simulink model "RC_buttom_Evaporator_1"  (R2018b)
settings: Solver=VariableStepAuto  StartTime=0.0  StopTime=500000.0  RelTol=1e-3
settings Model: Creator=user  LastModifiedBy=user

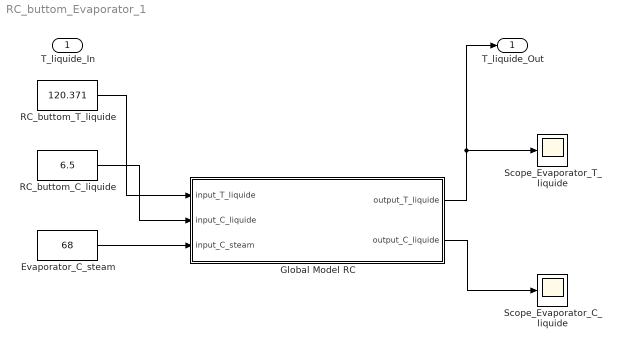
== system RC_buttom_Evaporator_1 ==
  T_liquide_In : Inport
  Evaporator_C_steam : Constant  Value=68
  Global Model RC : Subsystem
  RC_buttom_C_liquide : Constant  Value=6.5
  RC_buttom_T_liquide : Constant  Value=120.371
  Scope_Evaporator_C_liquide : Scope
  Scope_Evaporator_T_liquide : Scope
  T_liquide_Out : Outport
  wires:
  Global Model RC/1(output_T_liquide) -> T_liquide_Out/1, Scope_Evaporator_T_liquide/1
  Global Model RC/2(output_C_liquide) -> Scope_Evaporator_C_liquide/1
  Evaporator_C_steam/1 -> Global Model RC/3(input_C_steam)
  RC_buttom_C_liquide/1 -> Global Model RC/2(input_C_liquide)
  RC_buttom_T_liquide/1 -> Global Model RC/1(input_T_liquide)

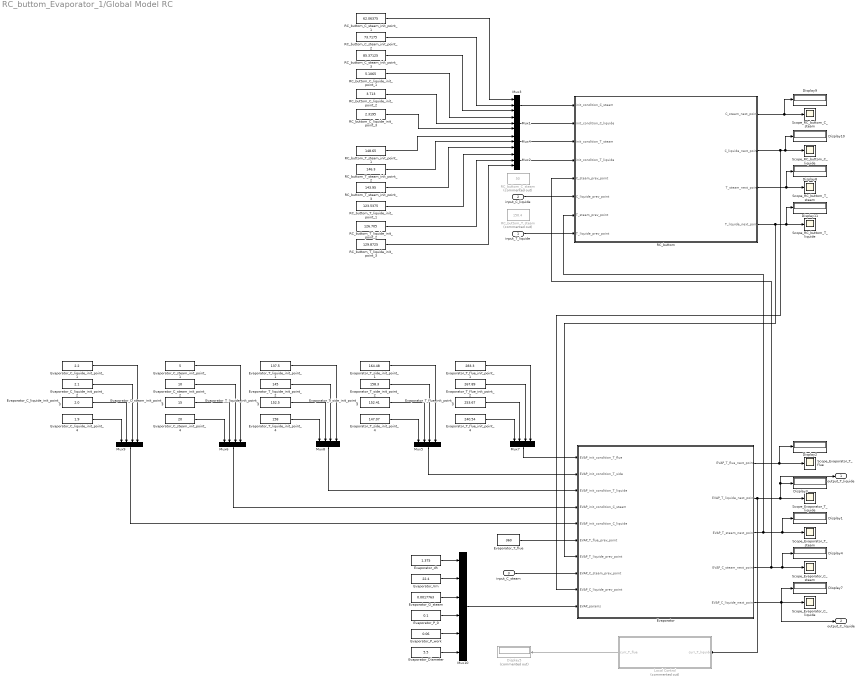
== system RC_buttom_Evaporator_1/Global Model RC ==
  input_T_liquide : Inport
  input_C_liquide : Inport  Port=2
  input_C_steam : Inport  Port=3
  Display{1..4,7..11} (9 alike) : Display
  Display5 : Display  Commented=on
  Evaporator : Subsystem
  Evaporator_C_liquide_init_point_1 : Constant  Value=2.2
  Evaporator_C_liquide_init_point_2 : Constant  Value=2.1
  Evaporator_C_liquide_init_point_3 : Constant  Value=2.0
  Evaporator_C_liquide_init_point_4 : Constant  Value=1.9
  Evaporator_C_steam_init_point_1 : Constant  Value=5
  Evaporator_C_steam_init_point_2 : Constant  Value=10
  Evaporator_C_steam_init_point_3 : Constant  Value=15
  Evaporator_C_steam_init_point_4 : Constant  Value=20
  Evaporator_Diameter : Constant  Value=5.5
  Evaporator_G_steam : Constant  Value=0.0017763
  Evaporator_P_0 : Constant  Value=0.1
  Evaporator_P_work : Constant  Value=0.06
  Evaporator_T_flue : Constant  Value=360
  Evaporator_T_flue_init_point_1 : Constant  Value=283.3
  Evaporator_T_flue_init_point_2 : Constant  Value=267.89
  Evaporator_T_flue_init_point_3 : Constant  Value=253.67
  Evaporator_T_flue_init_point_4 : Constant  Value=240.54
  Evaporator_T_liquide_init_point_1 : Constant  Value=137.5
  Evaporator_T_liquide_init_point_2 : Constant  Value=145
  Evaporator_T_liquide_init_point_3 : Constant  Value=152.5
  Evaporator_T_liquide_init_point_4 : Constant  Value=158
  Evaporator_T_side_init_point_1 : Constant  Value=164.48
  Evaporator_T_side_init_point_2 : Constant  Value=158.3
  Evaporator_T_side_init_point_3 : Constant  Value=152.41
  Evaporator_T_side_init_point_4 : Constant  Value=147.07
  Evaporator_Vm : Constant  Value=22.4
  Evaporator_dh : Constant  Value=1.375
  Local Control : Subsystem  Commented=on
  Mux{1..4} (4 alike) : Mux  Inputs=3
  Mux10 : Mux  Inputs=6
  Mux{5..9} (5 alike) : Mux
  RC_buttom : Subsystem
  RC_buttom_C_liquide_init_point_1 : Constant  Value=5.1065
  RC_buttom_C_liquide_init_point_2 : Constant  Value=3.713
  RC_buttom_C_liquide_init_point_3 : Constant  Value=2.3195
  RC_buttom_C_steam : Constant  Commented=on  Value=50
  RC_buttom_C_steam_init_point_1 : Constant  Value=62.06375
  RC_buttom_C_steam_init_point_2 : Constant  Value=73.7175
  RC_buttom_C_steam_init_point_3 : Constant  Value=85.37125
  RC_buttom_T_liquide_init_point_1 : Constant  Value=123.5375
  RC_buttom_T_liquide_init_point_2 : Constant  Value=126.705
  RC_buttom_T_liquide_init_point_3 : Constant  Value=129.8725
  RC_buttom_T_steam : Constant  Commented=on  Value=150.4
  RC_buttom_T_steam_init_point_1 : Constant  Value=148.65
  RC_buttom_T_steam_init_point_2 : Constant  Value=146.3
  RC_buttom_T_steam_init_point_3 : Constant  Value=143.95
  Scope_Evaporator_C_liquide : Scope
  Scope_Evaporator_C_steam : Scope
  Scope_Evaporator_T_flue : Scope
  Scope_Evaporator_T_liquide : Scope
  Scope_Evaporator_T_steam : Scope
  Scope_RC_buttom_C_liquide : Scope
  Scope_RC_buttom_C_steam : Scope
  Scope_RC_buttom_T_liquide : Scope
  Scope_RC_buttom_T_steam : Scope
  output_T_liquide : Outport
  output_C_liquide : Outport  Port=2
  wires:
  Evaporator_T_side_init_point_3/1 -> Mux5/2
  Evaporator_C_steam_init_point_2/1 -> Mux6/3
  Evaporator_C_liquide_init_point_1/1 -> Mux9/4
  RC_buttom_T_steam_init_point_1/1 -> Mux4/1
  Evaporator_C_steam_init_point_4/1 -> Mux6/1
  RC_buttom_C_steam_init_point_1/1 -> Mux3/1
  Mux1/1 -> RC_buttom/2(init_condition_C_liquide)
  Evaporator_T_liquide_init_point_4/1 -> Mux8/1
  Evaporator_C_steam_init_point_3/1 -> Mux6/2
  Evaporator/2(EVAP_T_liquide_next_point) -> Local Control/1(curr_T_liquide), output_T_liquide/1, Display3/1, Scope_Evaporator_T_liquide/1
  RC_buttom/4(T_liquide_next_point) -> Evaporator/7(EVAP_T_liquide_prev_point), Display11/1, Scope_RC_buttom_T_liquide/1
  Evaporator_C_liquide_init_point_2/1 -> Mux9/3
  Evaporator_G_steam/1 -> Mux10/3
  Local Control/1(curr_T_flue) -> Display5/1
  Mux8/1 -> Evaporator/3(EVAP_init_condition_T_liquide)
  Evaporator_P_0/1 -> Mux10/4
  Mux6/1 -> Evaporator/4(EVAP_init_condition_C_steam)
  Evaporator_T_flue_init_point_2/1 -> Mux7/3
  RC_buttom_C_liquide_init_point_2/1 -> Mux1/2
  Evaporator_P_work/1 -> Mux10/5
  RC_buttom_T_steam_init_point_3/1 -> Mux4/3
  Evaporator_C_liquide_init_point_3/1 -> Mux9/2
  Evaporator_C_liquide_init_point_4/1 -> Mux9/1
  input_T_liquide/1 -> RC_buttom/8(T_liquide_prev_point)
  Mux4/1 -> RC_buttom/3(init_condition_T_steam)
  Evaporator/1(EVAP_T_flue_next_point) -> Display2/1, Scope_Evaporator_T_flue/1
  Evaporator_T_flue_init_point_4/1 -> Mux7/1
  RC_buttom/3(T_steam_next_point) -> Display8/1, Scope_RC_buttom_T_steam/1
  Evaporator/3(EVAP_T_steam_next_point) -> Display1/1, Scope_Evaporator_T_steam/1, RC_buttom/7(T_steam_prev_point)
  RC_buttom_C_liquide_init_point_1/1 -> Mux1/1
  Evaporator_T_flue_init_point_1/1 -> Mux7/4
  RC_buttom/2(C_liquide_next_point) -> Display10/1, Scope_RC_buttom_C_liquide/1, Evaporator/9(EVAP_C_liquide_prev_point)
  Evaporator/5(EVAP_C_liquide_next_point) -> output_C_liquide/1, Display7/1, Scope_Evaporator_C_liquide/1
  Mux3/1 -> RC_buttom/1(init_condition_C_steam)
  Evaporator_T_side_init_point_1/1 -> Mux5/4
  RC_buttom_T_steam_init_point_2/1 -> Mux4/2
  RC_buttom_C_steam_init_point_2/1 -> Mux3/2
  Evaporator_T_side_init_point_2/1 -> Mux5/3
  RC_buttom_T_liquide_init_point_1/1 -> Mux2/1
  Evaporator_T_side_init_point_4/1 -> Mux5/1
  Evaporator_T_flue_init_point_3/1 -> Mux7/2
  RC_buttom_C_liquide_init_point_3/1 -> Mux1/3
  Evaporator_T_liquide_init_point_1/1 -> Mux8/4
  RC_buttom_T_liquide_init_point_3/1 -> Mux2/3
  RC_buttom/1(C_steam_next_point) -> Display9/1, Scope_RC_buttom_C_steam/1
  Evaporator_T_liquide_init_point_2/1 -> Mux8/3
  Evaporator_Vm/1 -> Mux10/2
  Mux7/1 -> Evaporator/1(EVAP_init_condition_T_flue)
  RC_buttom_T_liquide_init_point_2/1 -> Mux2/2
  Mux5/1 -> Evaporator/2(EVAP_init_condition_T_side)
  input_C_steam/1 -> Evaporator/8(EVAP_C_steam_prev_point)
  Mux2/1 -> RC_buttom/4(init_condition_T_liquide)
  Evaporator/4(EVAP_C_steam_next_point) -> RC_buttom/5(C_steam_prev_point), Display4/1, Scope_Evaporator_C_steam/1
  Mux10/1 -> Evaporator/10(EVAP_params)
  Evaporator_C_steam_init_point_1/1 -> Mux6/4
  Evaporator_T_liquide_init_point_3/1 -> Mux8/2
  Mux9/1 -> Evaporator/5(EVAP_init_condition_C_liquide)
  RC_buttom_C_steam_init_point_3/1 -> Mux3/3
  Evaporator_dh/1 -> Mux10/1
  Evaporator_Diameter/1 -> Mux10/6
  input_C_liquide/1 -> RC_buttom/6(C_liquide_prev_point)
  Evaporator_T_flue/1 -> Evaporator/6(EVAP_T_flue_prev_point)

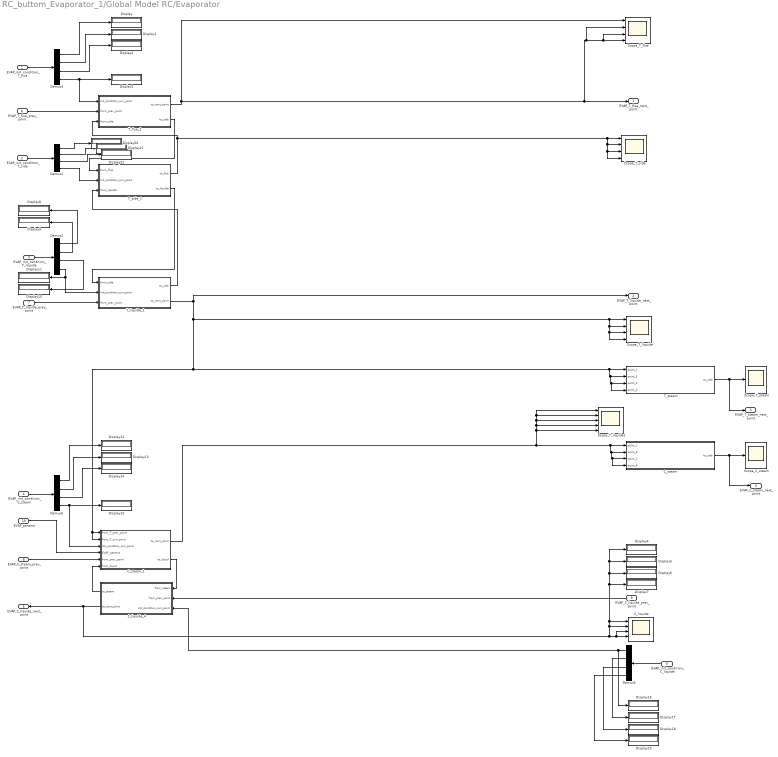
== system RC_buttom_Evaporator_1/Global Model RC/Evaporator ==
  EVAP_init_condition_T_flue : Inport
  EVAP_init_condition_T_side : Inport  Port=2
  EVAP_init_condition_T_liquide : Inport  Port=3
  EVAP_init_condition_C_steam : Inport  Port=4
  EVAP_init_condition_C_liquide : Inport  Port=5
  EVAP_T_flue_prev_point : Inport  Port=6
  EVAP_T_liquide_prev_point : Inport  Port=7
  EVAP_C_steam_prev_point : Inport  Port=8
  EVAP_C_liquide_prev_point : Inport  Port=9
  EVAP_params : Inport  Port=10
  C_liquide : Scope  NumInputPorts=4
  C_liquide_4 : Subsystem
  C_steam : Subsystem
  C_steam_1 : Subsystem
  Demux{1..5} (5 alike) : Demux
  Display{,1..22} (23 alike) : Display
  Scope_C_steam : Scope
  Scope_T_flue : Scope  NumInputPorts=4
  Scope_T_liquide : Scope  NumInputPorts=4
  Scope_T_liquide1 : Scope  NumInputPorts=5
  Scope_T_side : Scope  NumInputPorts=4
  Scope_T_steam : Scope
  T_flue_1 : Subsystem
  T_liquide_1 : Subsystem
  T_side_1 : Subsystem
  T_steam : Subsystem
  EVAP_T_flue_next_point : Outport
  EVAP_T_liquide_next_point : Outport  Port=2
  EVAP_T_steam_next_point : Outport  Port=3
  EVAP_C_steam_next_point : Outport  Port=4
  EVAP_C_liquide_next_point : Outport  Port=5
  wires:
  EVAP_init_condition_T_liquide/1 -> Demux2/1
  Demux2/1 -> Display8/1
  EVAP_init_condition_T_side/1 -> Demux1/1
  Demux2/2 -> Display9/1
  Demux2/4 -> T_liquide_1/2(init_condition_curr_point), Display11/1
  EVAP_init_condition_T_flue/1 -> Demux3/1
  Demux3/1 -> Display/1
  Demux3/2 -> Display1/1
  Demux3/3 -> Display2/1
  Demux3/4 -> T_flue_1/1(init_condition_curr_point), Display3/1
  T_flue_1/1(to_next_point) -> EVAP_T_flue_next_point/1, Scope_T_flue/2, Scope_T_flue/3, Scope_T_flue/4, Scope_T_flue/1
  EVAP_T_flue_prev_point/1 -> T_flue_1/2(from_prev_point)
  T_steam/1(to_side) -> EVAP_T_steam_next_point/1, Scope_T_steam/1
  Demux5/2 -> Display13/1
  EVAP_init_condition_C_liquide/1 -> Demux4/1
  Demux5/3 -> Display14/1
  C_steam_1/2(to_liquid) -> C_liquide_4/1(from_steam)
  Demux5/1 -> Display12/1
  EVAP_init_condition_C_steam/1 -> Demux5/1
  EVAP_C_steam_prev_point/1 -> C_steam_1/5(from_prev_point)
  C_liquide_4/2(to_next_point) -> EVAP_C_liquide_next_point/1, C_liquide/2, C_liquide/1, Display6/1, Display5/1, Display4/1, Display7/1, C_liquide/3, C_liquide/4
  EVAP_C_liquide_prev_point/1 -> C_liquide_4/2(from_prev_point)
  C_liquide_4/1(to_steam) -> C_steam_1/6(from_liquid)
  Demux5/4 -> C_steam_1/3(init_condition_curr_point), Display15/1
  Demux4/1 -> C_liquide_4/3(init_condition_curr_point), Display16/1
  Demux4/2 -> Display17/1
  Demux4/3 -> Display18/1
  Demux4/4 -> Display19/1
  C_steam/1(to_side) -> EVAP_C_steam_next_point/1, Scope_C_steam/1
  EVAP_params/1 -> C_steam_1/4(EVAP_params)
  EVAP_T_liquide_prev_point/1 -> T_liquide_1/3(from_prev_point)
  Demux2/3 -> Display10/1
  T_flue_1/2(to_side) -> T_side_1/1(from_flue)
  T_side_1/2(to_liquide) -> T_liquide_1/1(from_side)
  T_liquide_1/1(to_side) -> T_side_1/3(from_liquide)
  Demux1/4 -> T_side_1/2(init_condition_curr_point)
  T_side_1/1(to_flue) -> Scope_T_side/4, Scope_T_side/3, Scope_T_side/2, Scope_T_side/1, T_flue_1/3(from_side)
  Demux1/1 -> Display20/1
  Demux1/2 -> Display21/1
  Demux1/3 -> Display22/1
  T_liquide_1/2(to_next_point) -> EVAP_T_liquide_next_point/1, Scope_T_liquide/4, Scope_T_liquide/3, Scope_T_liquide/2, Scope_T_liquide/1, T_steam/4(point_4), T_steam/3(point_2), T_steam/2(point_3), T_steam/1(point_1), C_steam_1/1(from_T_prev_point), C_steam_1/2(from_T_curr_point)
  C_steam_1/1(to_next_point) -> Scope_T_liquide1/5, Scope_T_liquide1/4, Scope_T_liquide1/3, Scope_T_liquide1/2, Scope_T_liquide1/1, C_steam/4(point_4), C_steam/3(point_2), C_steam/2(point_3), C_steam/1(point_1)

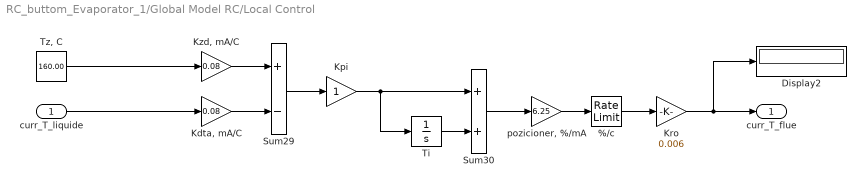
== system RC_buttom_Evaporator_1/Global Model RC/Local Control ==
  curr_T_liquide : Inport
  %/c : RateLimiter  RisingSlewLimit=5  FallingSlewLimit=-5  SampleTimeMode=inherited
  Display2 : Display
  "Kdta, mA/C" : Gain  Gain=0.08
  Kpi : Gain
  Kro : Gain  Gain=0.006
  "Kzd, mA/C" : Gain  Gain=0.08
  Sum29 : Sum  Inputs=+-
  Sum30 : Sum
  Ti : Integrator  InitialCondition=8000  UpperSaturationLimit=8012  LowerSaturationLimit=6012
  "Tz, C" : Constant  Value=160.00
  "pozicioner, %/mA" : Gain  Gain=6.25
  curr_T_flue : Outport
  wires:
  Ti/1 -> Sum30/2
  Kpi/1 -> Ti/1, Sum30/1
  "Tz, C"/1 -> "Kzd, mA/C"/1
  "Kzd, mA/C"/1 -> Sum29/1
  %/c/1 -> Kro/1
  "Kdta, mA/C"/1 -> Sum29/2
  curr_T_liquide/1 -> "Kdta, mA/C"/1
  "pozicioner, %/mA"/1 -> %/c/1
  Sum30/1 -> "pozicioner, %/mA"/1
  Kro/1 -> curr_T_flue/1, Display2/1
  Sum29/1 -> Kpi/1

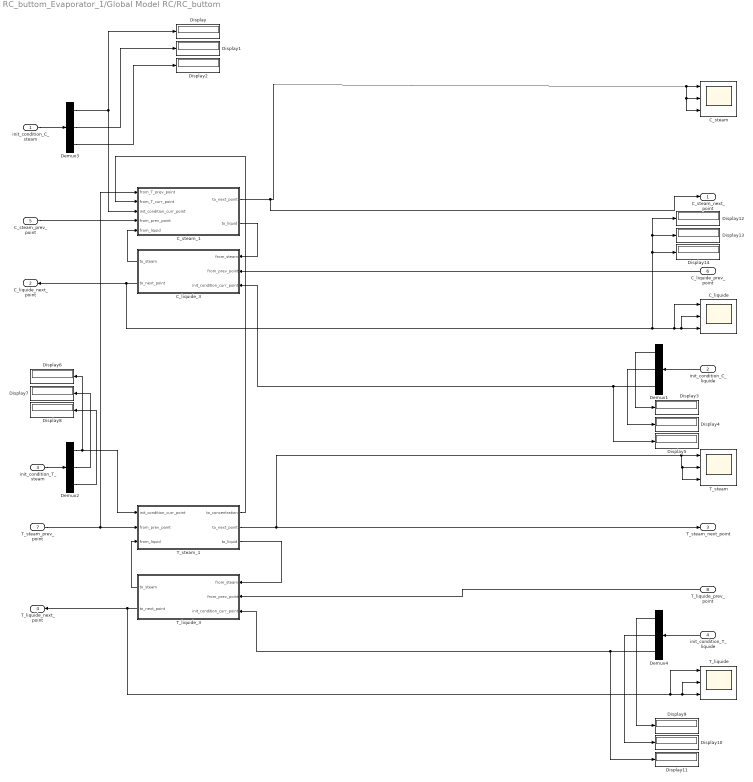
== system RC_buttom_Evaporator_1/Global Model RC/RC_buttom ==
  init_condition_C_steam : Inport
  init_condition_C_liquide : Inport  Port=2
  init_condition_T_steam : Inport  Port=3
  init_condition_T_liquide : Inport  Port=4
  C_steam_prev_point : Inport  Port=5
  C_liquide_prev_point : Inport  Port=6
  T_steam_prev_point : Inport  Port=7
  T_liquide_prev_point : Inport  Port=8
  C_liquide : Scope  NumInputPorts=3
  C_liquide_3 : Subsystem
  C_steam : Scope  NumInputPorts=3
  C_steam_1 : Subsystem
  Demux{1..4} (4 alike) : Demux  Outputs=3
  Display{,1..14} (15 alike) : Display
  T_liquide : Scope  NumInputPorts=3
  T_liquide_3 : Subsystem
  T_steam : Scope  NumInputPorts=3
  T_steam_1 : Subsystem
  C_steam_next_point : Outport
  C_liquide_next_point : Outport  Port=2
  T_steam_next_point : Outport  Port=3
  T_liquide_next_point : Outport  Port=4
  wires:
  T_steam_prev_point/1 -> C_steam_1/1(from_T_prev_point), T_steam_1/2(from_prev_point)
  T_liquide_prev_point/1 -> T_liquide_3/2(from_prev_point)
  T_steam_1/3(to_liquid) -> T_liquide_3/1(from_steam)
  T_liquide_3/1(to_steam) -> T_steam_1/3(from_liquid)
  Demux4/2 -> Display10/1
  Demux4/3 -> Display11/1, T_liquide_3/3(init_condition_curr_point)
  T_liquide_3/2(to_next_point) -> T_liquide/1, T_liquide/2, T_liquide/3, T_liquide_next_point/1
  C_liquide_3/1(to_steam) -> C_steam_1/5(from_liquid)
  C_steam_1/1(to_next_point) -> C_steam_next_point/1, C_steam/3, C_steam/2, C_steam/1
  Demux3/3 -> Display2/1
  C_liquide_prev_point/1 -> C_liquide_3/2(from_prev_point)
  C_liquide_3/2(to_next_point) -> Display12/1, Display13/1, Display14/1, C_liquide/1, C_liquide/2, C_liquide/3, C_liquide_next_point/1
  Demux1/2 -> Display4/1
  Demux1/3 -> C_liquide_3/3(init_condition_curr_point), Display5/1
  C_steam_prev_point/1 -> C_steam_1/4(from_prev_point)
  C_steam_1/2(to_liquid) -> C_liquide_3/1(from_steam)
  init_condition_T_steam/1 -> Demux2/1
  Demux2/1 -> T_steam_1/1(init_condition_curr_point), Display6/1
  Demux2/3 -> Display8/1
  init_condition_T_liquide/1 -> Demux4/1
  Demux4/1 -> Display9/1
  init_condition_C_steam/1 -> Demux3/1
  Demux3/2 -> Display1/1
  init_condition_C_liquide/1 -> Demux1/1
  Demux1/1 -> Display3/1
  Demux2/2 -> Display7/1
  Demux3/1 -> Display/1, C_steam_1/3(init_condition_curr_point)
  T_steam_1/1(to_concentration) -> C_steam_1/2(from_T_curr_point)
  T_steam_1/2(to_next_point) -> T_steam_next_point/1, T_steam/3, T_steam/2, T_steam/1

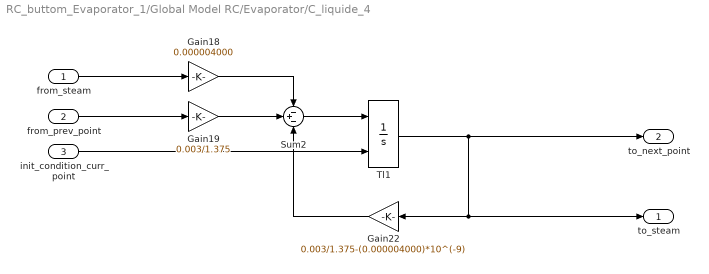
== system RC_buttom_Evaporator_1/Global Model RC/Evaporator/C_liquide_4 ==
  from_steam : Inport
  from_prev_point : Inport  Port=2
  init_condition_curr_point : Inport  Port=3
  Gain18 : Gain  Gain=0.000004000
  Gain19 : Gain  Gain=0.003/1.375
  Gain22 : Gain  Gain=0.003/1.375-(0.000004000)*10^(-9)
  Sum2 : Sum  Inputs=-+-
  Tl1 : Integrator  InitialConditionSource=external  InitialCondition=124.3766
  to_steam : Outport
  to_next_point : Outport  Port=2
  wires:
  from_steam/1 -> Gain18/1
  from_prev_point/1 -> Gain19/1
  Gain19/1 -> Sum2/2
  Sum2/1 -> Tl1/1
  Gain18/1 -> Sum2/1
  init_condition_curr_point/1 -> Tl1/2
  Gain22/1 -> Sum2/3
  Tl1/1 -> Gain22/1, to_steam/1, to_next_point/1

== system RC_buttom_Evaporator_1/Global Model RC/Evaporator/C_steam ==
  point_1 : Inport
  point_3 : Inport  Port=2
  point_2 : Inport  Port=3
  point_4 : Inport  Port=4
  Gain : Gain  Gain=1/4
  Sum37 : Sum  Inputs=++++
  to_side : Outport
  wires:
  point_2/1 -> Sum37/2
  point_1/1 -> Sum37/1
  point_3/1 -> Sum37/3
  point_4/1 -> Sum37/4
  Sum37/1 -> Gain/1
  Gain/1 -> to_side/1

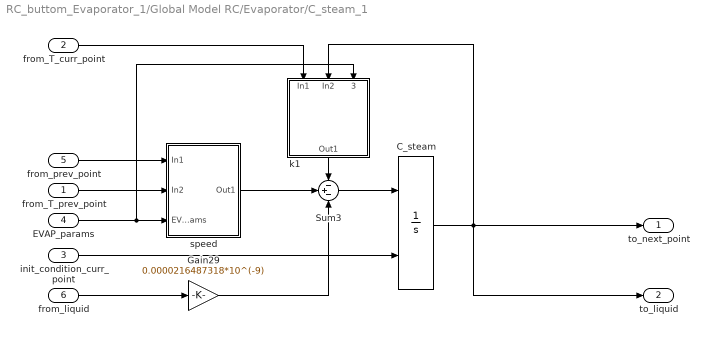
== system RC_buttom_Evaporator_1/Global Model RC/Evaporator/C_steam_1 ==
  from_T_prev_point : Inport
  from_T_curr_point : Inport  Port=2
  init_condition_curr_point : Inport  Port=3
  EVAP_params : Inport  Port=4
  from_prev_point : Inport  Port=5
  from_liquid : Inport  Port=6
  C_steam : Integrator  InitialConditionSource=external  InitialCondition=156.9966
  Gain29 : Gain  Gain=0.0000216487318*10^(-9)
  Sum3 : Sum  Inputs=-+-
  k1 : Subsystem
  speed : Subsystem
  to_next_point : Outport
  to_liquid : Outport  Port=2
  wires:
  init_condition_curr_point/1 -> C_steam/2
  speed/1(Out1) -> Sum3/2
  Gain29/1 -> Sum3/3
  Sum3/1 -> C_steam/1
  from_liquid/1 -> Gain29/1
  k1/1(Out1) -> Sum3/1
  C_steam/1 -> k1/2(In2), to_next_point/1, to_liquid/1
  from_T_curr_point/1 -> k1/1(In1)
  EVAP_params/1 -> k1/3(EVAP_params1), speed/3(EVAP_params)
  from_prev_point/1 -> speed/1(In1)
  from_T_prev_point/1 -> speed/2(In2)

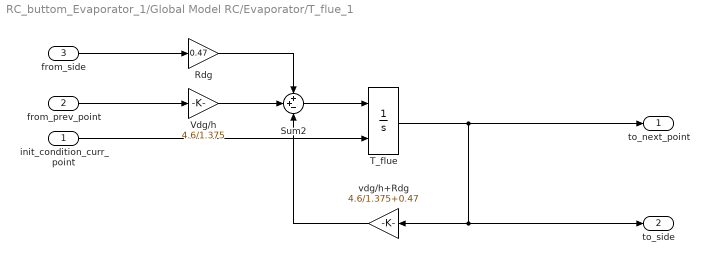
== system RC_buttom_Evaporator_1/Global Model RC/Evaporator/T_flue_1 ==
  init_condition_curr_point : Inport
  from_prev_point : Inport  Port=2
  from_side : Inport  Port=3
  Rdg : Gain  Gain=0.47
  Sum2 : Sum  Inputs=++-
  T_flue : Integrator  InitialConditionSource=external  InitialCondition=124.3766
  Vdg/h : Gain  Gain=4.6/1.375
  vdg/h+Rdg : Gain  Gain=4.6/1.375+0.47
  to_next_point : Outport
  to_side : Outport  Port=2
  wires:
  Vdg/h/1 -> Sum2/2
  from_prev_point/1 -> Vdg/h/1
  from_side/1 -> Rdg/1
  vdg/h+Rdg/1 -> Sum2/3
  Sum2/1 -> T_flue/1
  Rdg/1 -> Sum2/1
  init_condition_curr_point/1 -> T_flue/2
  T_flue/1 -> to_next_point/1, vdg/h+Rdg/1, to_side/1

== system RC_buttom_Evaporator_1/Global Model RC/Evaporator/T_liquide_1 ==
  from_side : Inport
  init_condition_curr_point : Inport  Port=2
  from_prev_point : Inport  Port=3
  Ra : Gain  Gain=0.003
  Sum37 : Sum  Inputs=++-
  T_liquide : Integrator  InitialConditionSource=external  InitialCondition=136.285
  va/h+Ra : Gain  Gain=0.003/1.375+0.003
  va/h1 : Gain  Gain=0.003/1.375
  to_side : Outport
  to_next_point : Outport  Port=2
  wires:
  init_condition_curr_point/1 -> T_liquide/2
  va/h1/1 -> Sum37/2
  Sum37/1 -> T_liquide/1
  from_prev_point/1 -> va/h1/1
  Ra/1 -> Sum37/1
  from_side/1 -> Ra/1
  T_liquide/1 -> to_next_point/1, va/h+Ra/1, to_side/1
  va/h+Ra/1 -> Sum37/3

== system RC_buttom_Evaporator_1/Global Model RC/Evaporator/T_side_1 ==
  from_flue : Inport
  init_condition_curr_point : Inport  Port=2
  from_liquide : Inport  Port=3
  Rast : Gain  Gain=0.22
  Rdgst : Gain  Gain=0.008
  Rdgst+Rast : Gain  Gain=0.008+0.22
  Sum2 : Sum  Inputs=++-
  T_side : Integrator  InitialConditionSource=external  InitialCondition=124.3766
  to_flue : Outport
  to_liquide : Outport  Port=2
  wires:
  Rast/1 -> Sum2/2
  from_liquide/1 -> Rast/1
  from_flue/1 -> Rdgst/1
  T_side/1 -> Rdgst+Rast/1, to_liquide/1, to_flue/1
  Rdgst+Rast/1 -> Sum2/3
  Sum2/1 -> T_side/1
  Rdgst/1 -> Sum2/1
  init_condition_curr_point/1 -> T_side/2

== system RC_buttom_Evaporator_1/Global Model RC/Evaporator/T_steam ==
  point_1 : Inport
  point_3 : Inport  Port=2
  point_2 : Inport  Port=3
  point_4 : Inport  Port=4
  Gain : Gain  Gain=1/4
  Sum37 : Sum  Inputs=++++
  to_side : Outport
  wires:
  point_2/1 -> Sum37/2
  point_1/1 -> Sum37/1
  point_3/1 -> Sum37/3
  point_4/1 -> Sum37/4
  Sum37/1 -> Gain/1
  Gain/1 -> to_side/1

== system RC_buttom_Evaporator_1/Global Model RC/RC_buttom/C_liquide_3 ==
  from_steam : Inport
  from_prev_point : Inport  Port=2
  init_condition_curr_point : Inport  Port=3
  Gain18 : Gain  Gain=0.000010734
  Gain19 : Gain  Gain=0.0002291314/0.5
  Gain22 : Gain  Gain=0.0002291314/0.5-(0.000010734)*10^(-9)
  Sum2 : Sum  Inputs=-+-
  Tl1 : Integrator  InitialConditionSource=external  InitialCondition=124.3766
  to_steam : Outport
  to_next_point : Outport  Port=2
  wires:
  Gain22/1 -> Sum2/3
  Gain19/1 -> Sum2/2
  Sum2/1 -> Tl1/1
  Tl1/1 -> Gain22/1, to_steam/1, to_next_point/1
  Gain18/1 -> Sum2/1
  init_condition_curr_point/1 -> Tl1/2
  from_prev_point/1 -> Gain19/1
  from_steam/1 -> Gain18/1

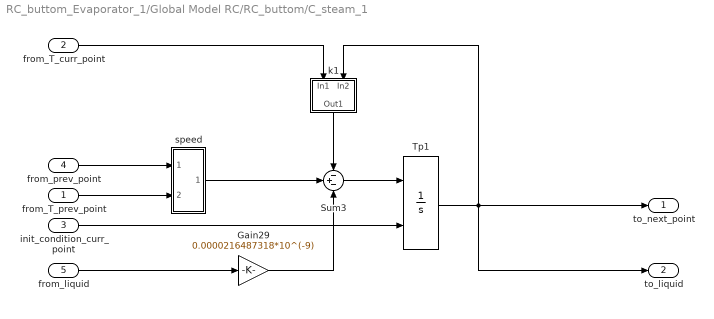
== system RC_buttom_Evaporator_1/Global Model RC/RC_buttom/C_steam_1 ==
  from_T_prev_point : Inport
  from_T_curr_point : Inport  Port=2
  init_condition_curr_point : Inport  Port=3
  from_prev_point : Inport  Port=4
  from_liquid : Inport  Port=5
  Gain29 : Gain  Gain=0.0000216487318*10^(-9)
  Sum3 : Sum  Inputs=-+-
  Tp1 : Integrator  InitialConditionSource=external  InitialCondition=156.9966
  k1 : Subsystem
  speed : Subsystem
  to_next_point : Outport
  to_liquid : Outport  Port=2
  wires:
  init_condition_curr_point/1 -> Tp1/2
  speed/1(Out1) -> Sum3/2
  Gain29/1 -> Sum3/3
  Sum3/1 -> Tp1/1
  from_liquid/1 -> Gain29/1
  k1/1(Out1) -> Sum3/1
  Tp1/1 -> k1/2(In2), to_next_point/1, to_liquid/1
  from_T_curr_point/1 -> k1/1(In1)
  from_T_prev_point/1 -> speed/2(In2)
  from_prev_point/1 -> speed/1(In1)

== system RC_buttom_Evaporator_1/Global Model RC/RC_buttom/T_liquide_3 ==
  from_steam : Inport
  from_prev_point : Inport  Port=2
  init_condition_curr_point : Inport  Port=3
  Gain4 : Gain  Gain=0.0000777
  Gain5 : Gain  Gain=0.0002291314/0.5
  Gain8 : Gain  Gain=0.0002291314/0.5+0.0000777
  Sum2 : Sum  Inputs=++-
  Tl1 : Integrator  InitialConditionSource=external  InitialCondition=124.3766
  to_steam : Outport
  to_next_point : Outport  Port=2
  wires:
  from_prev_point/1 -> Gain5/1
  Gain4/1 -> Sum2/1
  Tl1/1 -> to_steam/1, Gain8/1, to_next_point/1
  Gain8/1 -> Sum2/3
  Gain5/1 -> Sum2/2
  from_steam/1 -> Gain4/1
  init_condition_curr_point/1 -> Tl1/2
  Sum2/1 -> Tl1/1

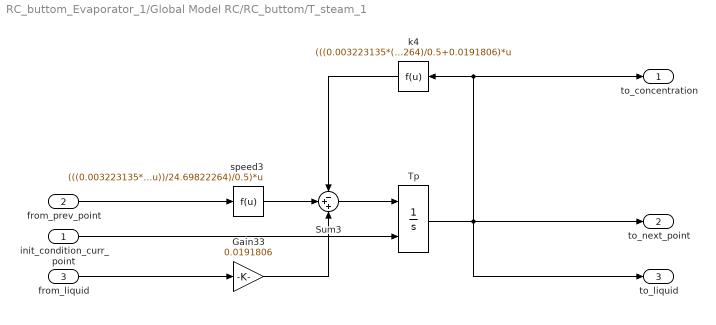
== system RC_buttom_Evaporator_1/Global Model RC/RC_buttom/T_steam_1 ==
  init_condition_curr_point : Inport
  from_prev_point : Inport  Port=2
  from_liquid : Inport  Port=3
  Gain33 : Gain  Gain=0.0191806
  Sum3 : Sum  Inputs=-++
  Tp : Integrator  InitialConditionSource=external  InitialCondition=156.9966
  k4 : Fcn  Expr=(((0.003223135*(273+u))/24.69822264)/0.5+0.0191806)*u
  speed3 : Fcn  Expr=(((0.003223135*(273+u))/24.69822264)/0.5)*u
  to_concentration : Outport
  to_next_point : Outport  Port=2
  to_liquid : Outport  Port=3
  wires:
  init_condition_curr_point/1 -> Tp/2
  speed3/1 -> Sum3/2
  Gain33/1 -> Sum3/3
  Sum3/1 -> Tp/1
  from_prev_point/1 -> speed3/1
  k4/1 -> Sum3/1
  from_liquid/1 -> Gain33/1
  Tp/1 -> k4/1, to_concentration/1, to_next_point/1, to_liquid/1

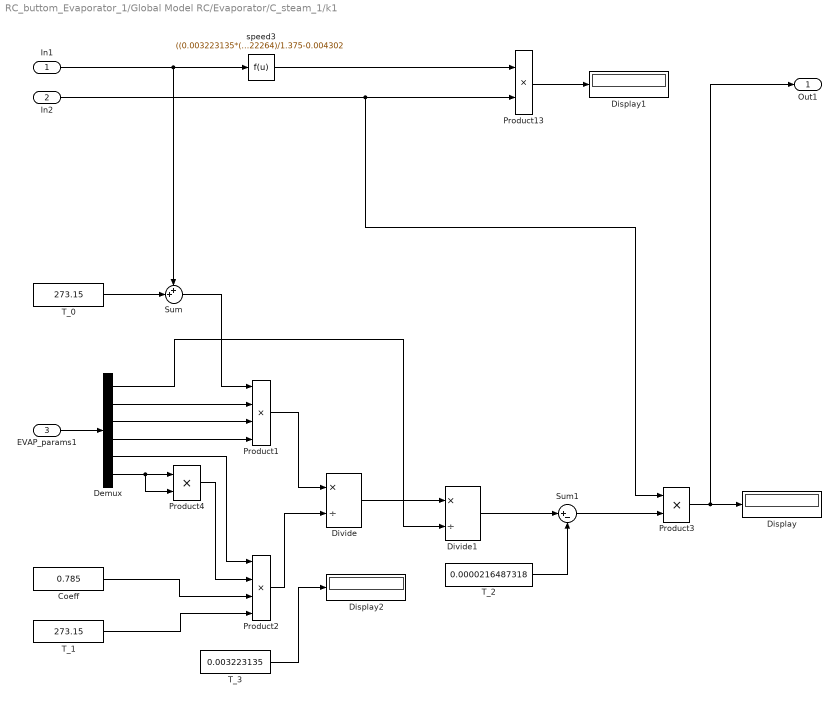
== system RC_buttom_Evaporator_1/Global Model RC/Evaporator/C_steam_1/k1 ==
  In1 : Inport
  In2 : Inport  Port=2
  EVAP_params1 : Inport  Port=3
  Coeff : Constant  Value=0.785
  Demux : Demux  Outputs=6
  Display : Display
  Display1 : Display
  Display2 : Display
  Divide : Product  Inputs=*/
  Divide1 : Product  Inputs=*/
  Product1 : Product  Inputs=4  SaturateOnIntegerOverflow=on  InputSameDT=on  OutDataTypeStr=Inherit: Same as first input
  Product13 : Product  SaturateOnIntegerOverflow=on  InputSameDT=on  OutDataTypeStr=Inherit: Same as first input
  Product2 : Product  Inputs=4  SaturateOnIntegerOverflow=on  InputSameDT=on  OutDataTypeStr=Inherit: Same as first input
  Product3 : Product  SaturateOnIntegerOverflow=on  InputSameDT=on  OutDataTypeStr=Inherit: Same as first input
  Product4 : Product  SaturateOnIntegerOverflow=on  InputSameDT=on  OutDataTypeStr=Inherit: Same as first input
  Sum : Sum  Inputs=++|
  Sum1 : Sum  Inputs=|+-
  T_0 : Constant  Value=273.15
  T_1 : Constant  Value=273.15
  T_2 : Constant  Value=0.0000216487318
  T_3 : Constant  Value=0.003223135
  speed3 : Fcn  Expr=((0.003223135*(273+u))/24.69822264)/1.375-0.004302
  Out1 : Outport
  wires:
  speed3/1 -> Product13/1
  T_1/1 -> Product2/4
  Divide/1 -> Divide1/1
  EVAP_params1/1 -> Demux/1
  Demux/1 -> Divide1/2
  Demux/6 -> Product4/2, Product4/1
  In2/1 -> Product3/1, Product13/2
  Coeff/1 -> Product2/3
  In1/1 -> Sum/1, speed3/1
  Demux/4 -> Product1/4
  Demux/5 -> Product2/1
  Demux/3 -> Product1/3
  Product4/1 -> Product2/2
  Product3/1 -> Out1/1, Display/1
  T_0/1 -> Sum/2
  Product1/1 -> Divide/1
  Sum/1 -> Product1/1
  Demux/2 -> Product1/2
  Product13/1 -> Display1/1
  Sum1/1 -> Product3/2
  Divide1/1 -> Sum1/1
  T_2/1 -> Sum1/2
  T_3/1 -> Display2/1
  Product2/1 -> Divide/2

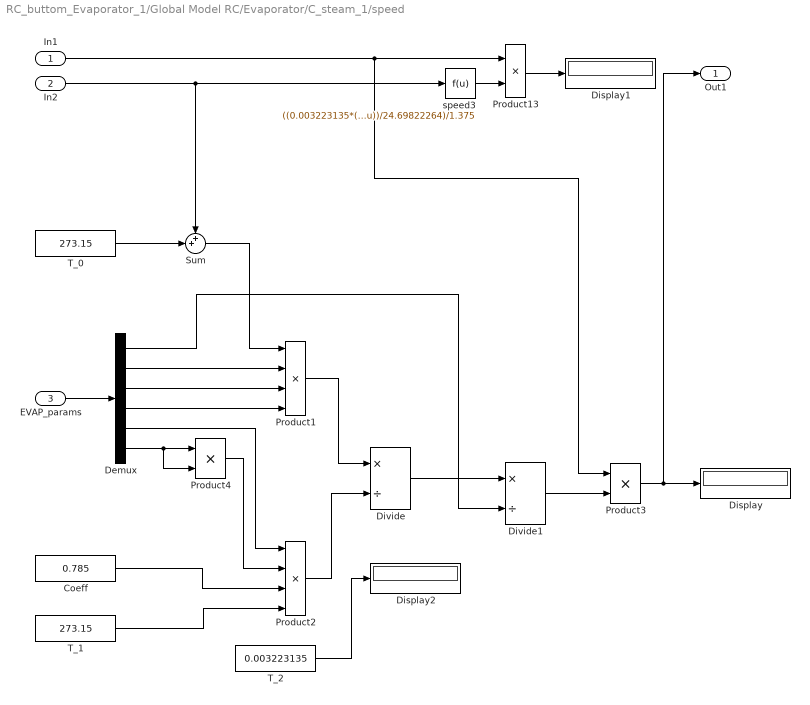
== system RC_buttom_Evaporator_1/Global Model RC/Evaporator/C_steam_1/speed ==
  In1 : Inport
  In2 : Inport  Port=2
  EVAP_params : Inport  Port=3
  Coeff : Constant  Value=0.785
  Demux : Demux  Outputs=6
  Display : Display
  Display1 : Display
  Display2 : Display
  Divide : Product  Inputs=*/
  Divide1 : Product  Inputs=*/
  Product1 : Product  Inputs=4  SaturateOnIntegerOverflow=on  InputSameDT=on  OutDataTypeStr=Inherit: Same as first input
  Product13 : Product  SaturateOnIntegerOverflow=on  InputSameDT=on  OutDataTypeStr=Inherit: Same as first input
  Product2 : Product  Inputs=4  SaturateOnIntegerOverflow=on  InputSameDT=on  OutDataTypeStr=Inherit: Same as first input
  Product3 : Product  SaturateOnIntegerOverflow=on  InputSameDT=on  OutDataTypeStr=Inherit: Same as first input
  Product4 : Product  SaturateOnIntegerOverflow=on  InputSameDT=on  OutDataTypeStr=Inherit: Same as first input
  Sum : Sum  Inputs=++|
  T_0 : Constant  Value=273.15
  T_1 : Constant  Value=273.15
  T_2 : Constant  Value=0.003223135
  speed3 : Fcn  Expr=((0.003223135*(273+u))/24.69822264)/1.375
  Out1 : Outport
  wires:
  In1/1 -> Product3/1, Product13/1
  In2/1 -> Sum/1, speed3/1
  speed3/1 -> Product13/2
  EVAP_params/1 -> Demux/1
  Demux/2 -> Product1/2
  Demux/3 -> Product1/3
  Demux/4 -> Product1/4
  Sum/1 -> Product1/1
  T_0/1 -> Sum/2
  Demux/5 -> Product2/1
  Coeff/1 -> Product2/3
  T_1/1 -> Product2/4
  Product1/1 -> Divide/1
  Product2/1 -> Divide/2
  Divide/1 -> Divide1/1
  Demux/1 -> Divide1/2
  Divide1/1 -> Product3/2
  Demux/6 -> Product4/2, Product4/1
  Product4/1 -> Product2/2
  Product3/1 -> Out1/1, Display/1
  Product13/1 -> Display1/1
  T_2/1 -> Display2/1

== system RC_buttom_Evaporator_1/Global Model RC/RC_buttom/C_steam_1/k1 ==
  In1 : Inport
  In2 : Inport  Port=2
  Product13 : Product  SaturateOnIntegerOverflow=on  InputSameDT=on  OutDataTypeStr=Inherit: Same as first input
  speed3 : Fcn  Expr=((0.003223135*(273+u))/24.69822264)/0.5-0.0000216487318
  Out1 : Outport
  wires:
  Product13/1 -> Out1/1
  speed3/1 -> Product13/1
  In1/1 -> speed3/1
  In2/1 -> Product13/2

== system RC_buttom_Evaporator_1/Global Model RC/RC_buttom/C_steam_1/speed ==
  In1 : Inport
  In2 : Inport  Port=2
  Product13 : Product  SaturateOnIntegerOverflow=on  InputSameDT=on  OutDataTypeStr=Inherit: Same as first input
  speed3 : Fcn  Expr=((0.003223135*(273+u))/24.69822264)/0.5
  Out1 : Outport
  wires:
  In1/1 -> Product13/1
  In2/1 -> speed3/1
  speed3/1 -> Product13/2
  Product13/1 -> Out1/1
